simulink model "QuadrotorSimulink_no_memory"  (R2020a)
settings: Solver=FixedStepAuto  StartTime=0.0  StopTime=options.T_train  FixedStep=options.dt  RelTol=1e-6
undefined symbols (not defined in the file or in its folder): options, Quad
libraries: neural x67, simulink x1
(part 4 of 4)

== system QuadrotorSimulink_no_memory/NN/Layer 3/Delays 1 ==
  "p{3}" : Inport  PortDimensions=30
      mask Display: e = 0.06;c1 = [120 230 180]/255;c2 = ([120 230 180]+0)/(256+128);c3 = ([120 230 180]+128)/(256+128);patch([0 1 1 0],[0 0 1 1],c1);patch([0 1 1 1-e 1-e 0+e],[0 0 1 1-e 0+e 0+e],c2);patch([0 0 1 1-e 0+e 0+e],[0 1 1 1-e 1-e 0+e],c3);plot([0 1 1 0 0],[0 0 1 1 0]);
  mux : Mux  Inputs=1
      mask Display: e = 0.06;c1 = [120 150 230]/255;c2 = ([120 150 230]+0)/383;c3 = ([120 150 230]+128)/383;patch([0 1 1 0],[0 0 1 1],c1);patch([0 1 1 1-e 1-e 0+e],[0 0 1 1-e 0+e 0+e],c2);patch([0 0 1 1-e 0+e 0+e],[0 1 1 1-e 1-e 0+e],c3);plot([0 1 1 0 0],[0 0 1 1 0]);disp('Mux')
  "pd{3,2}" : Outport
      mask Display: e = 0.06;c1 = [120 230 180]/255;c2 = ([120 230 180]+0)/(256+128);c3 = ([120 230 180]+128)/(256+128);patch([0 1 1 0],[0 0 1 1],c1);patch([0 1 1 1-e 1-e 0+e],[0 0 1 1-e 0+e 0+e],c2);patch([0 0 1 1-e 0+e 0+e],[0 1 1 1-e 1-e 0+e],c3);plot([0 1 1 0 0],[0 0 1 1 0]);
  wires:
  "p{3}"/1 -> mux/1
  mux/1 -> "pd{3,2}"/1

== system QuadrotorSimulink_no_memory/NN/Layer 3/LW{3,2} ==
  "ad{3,2}" : Inport  PortDimensions=30
      mask Display: e = 0.06;c1 = [120 230 180]/255;c2 = ([120 230 180]+0)/(256+128);c3 = ([120 230 180]+128)/(256+128);patch([0 1 1 0],[0 0 1 1],c1);patch([0 1 1 1-e 1-e 0+e],[0 0 1 1-e 0+e 0+e],c2);patch([0 0 1 1-e 0+e 0+e],[0 1 1 1-e 1-e 0+e],c3);plot([0 1 1 0 0],[0 0 1 1 0]);
  "IW{3,2}(1,:)'" : Constant  Value=[-0.89718489983829752265620527396094985306262969970703125;-1.2148392043519102845294810322229750454425811767578125;0.56509166986029313317629885204951278865337371826171875;-1.1504170795476256206057996678282506763935089111328125;1.487683784925635688267675504903309047222137451171875;0.18665373094955561850127878642524592578411102294921875;0.62008627570132446304995710306684486567974090576171875;1.55757000242328302874739165417850017547607421875;-1.9707156638451508445797344393213279545307159423828125;-1.2706500720731532805274355268920771777629852294921875;-0.2167436242368831755822355944474111311137676239013671875;-1.1468899065923487956553117328439839184284210205078125;1.0110761561406409470009748474694788455963134765625;-0.84398151321046521733393319664173759520053863525390625;-0.1453665614117256310588999212995986454188823699951171875;-1.076141234189552875477602356113493442535400390625;1.5832415842938474259682379852165468037128448486328125;1.33259473389290139522245226544328033924102783203125;-1.1165024930535540903520086430944502353668212890625;-0.780360767588013093387644403264857828617095947265625;1.2840319129847277412892481152084656059741973876953125;0.41948967045633078765121126707526855170726776123046875;-0.1531891438920943981916167331291944719851016998291015625;-0.817618197687156378350437080371193587779998779296875;1.780410080625970170586924723465926945209503173828125;1.7297582828772506413628207155852578580379486083984375;0.99332755179906973008741033481783233582973480224609375;0.3131520372519747130723999362089671194553375244140625;1.1515249808260035191409542676410637795925140380859375;1.7946714550899798279459673722158186137676239013671875]
      mask Display: e = 0.06;c1 = [120 150 230]/255;c2 = ([120 150 230]+0)/383;c3 = ([120 150 230]+128)/383;patch([0 1 1 0],[0 0 1 1],c1);patch([0 1 1 1-e 1-e 0+e],[0 0 1 1-e 0+e 0+e],c2);patch([0 0 1 1-e 0+e 0+e],[0 1 1 1-e 1-e 0+e],c3);plot([0 1 1 0 0],[0 0 1 1 0]);disp('weights');
  "IW{3,2}(2,:)'" : Constant  Value=[-0.1878719191598685334110285793940420262515544891357421875;0.401490952862056771355270257117808796465396881103515625;0.72936134659137008551255121346912346780300140380859375;-0.0102259523590943028625854793745020288042724132537841796875;-0.4768124734760250671428138957708142697811126708984375;0.3808058389067088267410099433618597686290740966796875;-0.66426163139011029645786265973583795130252838134765625;-0.614651116235851002755907757091335952281951904296875;0.552141523195427641468313595396466553211212158203125;0.4867297308495410756989940637140534818172454833984375;-0.081545652512581778825762057749670930206775665283203125;0.306546683783301687764577536654542200267314910888671875;-0.1636747505705764549333025570376776158809661865234375;0.4889788867021744867003008039318956434726715087890625;0.469842897528570391241231618550955317914485931396484375;0.389098199752417828189976489738910458981990814208984375;0.110536569007330387481857769671478308737277984619140625;-0.476156056619628176296288302182801999151706695556640625;0.41343160978527893067990817144163884222507476806640625;0.6146374534580640869307899265550076961517333984375;-0.08482317907464197170863684505093260668218135833740234375;0.61400646630597766062464870628900825977325439453125;-0.18723128910665132185187076174770481884479522705078125;0.07272131090734833269717540815690881572663784027099609375;-0.704997395230613665972896342282183468341827392578125;-0.442244488710228977890182022747467271983623504638671875;-0.1552661024650533183599776521077728830277919769287109375;0.70615630498671821957401562031009234488010406494140625;-0.38704845081048333543805028966744430363178253173828125;-0.45454456083797112331268408524920232594013214111328125]
      mask Display: e = 0.06;c1 = [120 150 230]/255;c2 = ([120 150 230]+0)/383;c3 = ([120 150 230]+128)/383;patch([0 1 1 0],[0 0 1 1],c1);patch([0 1 1 1-e 1-e 0+e],[0 0 1 1-e 0+e 0+e],c2);patch([0 0 1 1-e 0+e 0+e],[0 1 1 1-e 1-e 0+e],c3);plot([0 1 1 0 0],[0 0 1 1 0]);disp('weights');
  Mux : Mux  Inputs=2
      mask Display: e = 0.06;c1 = [120 150 230]/255;c2 = ([120 150 230]+0)/383;c3 = ([120 150 230]+128)/383;patch([0 1 1 0],[0 0 1 1],c1);patch([0 1 1 1-e 1-e 0+e],[0 0 1 1-e 0+e 0+e],c2);patch([0 0 1 1-e 0+e 0+e],[0 1 1 1-e 1-e 0+e],c3);plot([0 1 1 0 0],[0 0 1 1 0]);disp('Mux');
  dotprod1 : neural/Weight Functions/dotprod
  dotprod2 : neural/Weight Functions/dotprod
  "lz{3,2}" : Outport
      mask Display: e = 0.06;c1 = [120 230 180]/255;c2 = ([120 230 180]+0)/(256+128);c3 = ([120 230 180]+128)/(256+128);patch([0 1 1 0],[0 0 1 1],c1);patch([0 1 1 1-e 1-e 0+e],[0 0 1 1-e 0+e 0+e],c2);patch([0 0 1 1-e 0+e 0+e],[0 1 1 1-e 1-e 0+e],c3);plot([0 1 1 0 0],[0 0 1 1 0]);
  wires:
  "IW{3,2}(1,:)'"/1 -> dotprod1/1
  "ad{3,2}"/1 -> dotprod1/2, dotprod2/2
  dotprod1/1 -> Mux/1
  "IW{3,2}(2,:)'"/1 -> dotprod2/1
  dotprod2/1 -> Mux/2
  Mux/1 -> "lz{3,2}"/1
